simulink model "chap10_2sim"  (R2015a)
settings: Solver=ode45  StartTime=0.0  StopTime=40  RelTol=1e-3
settings Model: Creator=zhr  LastModifiedBy=IT

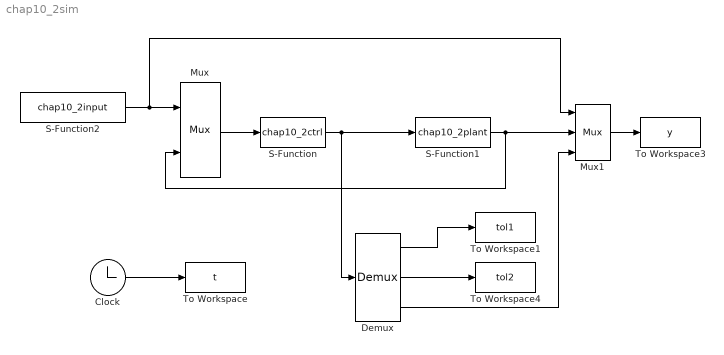
== system chap10_2sim ==
  Clock : Clock
  Demux : Demux  Outputs=3
  Mux : Mux  Inputs=2
  Mux1 : Mux  Inputs=3
  S-Function : S-Function  FunctionName=chap10_2ctrl
  S-Function1 : S-Function  FunctionName=chap10_2plant
  S-Function2 : S-Function  FunctionName=chap10_2input
  To Workspace : ToWorkspace  VariableName=t  SampleTime=-1
  To Workspace1 : ToWorkspace  VariableName=tol1  SampleTime=-1
  To Workspace3 : ToWorkspace  VariableName=y  SampleTime=-1
  To Workspace4 : ToWorkspace  VariableName=tol2  SampleTime=-1
  wires:
  Clock/1 -> To Workspace/1
  S-Function2/1 -> Mux/1, Mux1/1
  Mux/1 -> S-Function/1
  S-Function/1 -> Demux/1, S-Function1/1
  Demux/1 -> To Workspace1/1
  S-Function1/1 -> Mux1/2, Mux/2
  Mux1/1 -> To Workspace3/1
  Demux/2 -> To Workspace4/1
  Demux/3 -> Mux1/3
